simulink model "teste2"  (R2017a)
settings: Solver=VariableStepAuto  StartTime=0.0  StopTime=10.0  RelTol=1e-3
settings Model: Creator=felip  LastModifiedBy=felip

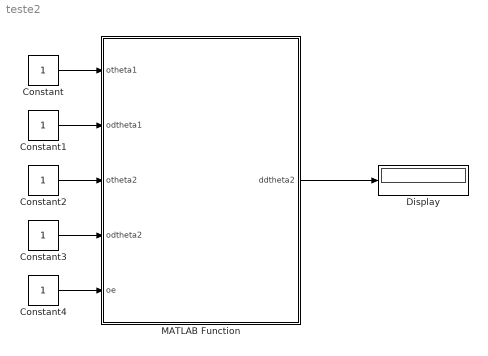
== system teste2 ==
  Constant{,1..4} (5 alike) : Constant
  Display : Display
  MATLAB Function : MATLAB Function  TreatAsAtomicUnit=on
  wires:
  Constant1/1 -> MATLAB Function/2(odtheta1)
  Constant/1 -> MATLAB Function/1(otheta1)
  Constant4/1 -> MATLAB Function/5(oe)
  Constant3/1 -> MATLAB Function/4(odtheta2)
  Constant2/1 -> MATLAB Function/3(otheta2)
  MATLAB Function/1(ddtheta2) -> Display/1

== matlab function teste2/MATLAB Function ==
  data: otheta1 input; ddtheta2 output; odtheta1 input; otheta2 input; odtheta2 input; oe input
function ddtheta2 = fcn2(otheta1,odtheta1,otheta2,odtheta2,oe)

ddtheta2 = zeros(1,1);  
coder.extrinsic('syms')
coder.extrinsic('symfun')
syms theta1 dtheta1 theta2 dtheta2 e;
Func2=symfun((1536877429000564048815928821109619140625*dtheta2 - 78627156504041188505523135421261472071680000*sin(theta2) - 634916175454785429479332065228843667947520*dtheta1^2*sin(2*theta2) + 79739804918975647357573983605853100441600*dtheta2^2*sin(2*theta2) + 3215150499355185931248636722272000000000*dtheta1*cos(theta2) - 2329329519919803072008927828125000000000*e*cos(theta2) - 4488271131060137965939268641213019848704000*sin(theta2)*(sin(theta2)^2 - 1) - 87729518696337784553411358347656250000*dtheta2*cos(theta2)^2 + 215034938293347338563840361500378723778560*dtheta1*dtheta2*(sin(theta2) - sin(theta2)^3) + 72485794161724834273391887682518082650112*dtheta1^2*cos(theta2)^3*sin(theta2))/(5575456338684674048*(41721610581794358547444*cos(theta2)^2 - 229801380526943752815105)),[theta1 dtheta1 theta2 dtheta2 e])
ddtheta2 = vpa(subs(Func2,[theta1 dtheta1 theta2 dtheta2 e],[odtheta1,otheta1,odtheta2,otheta2,oe]));
